simulink model "untitled1"  (R2023a)
settings: Solver=VariableStepAuto  StartTime=0.0  StopTime=30  RelTol=1e-3
settings Model: Creator=Sumeadh  LastModifiedBy=Sumeadh

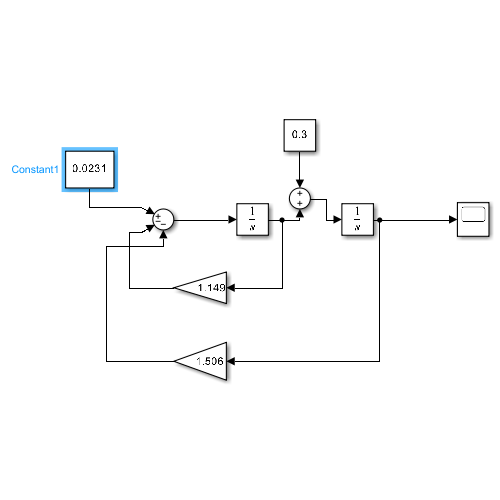
[thumbnail: Simulink's stored preview of the top-level diagram]
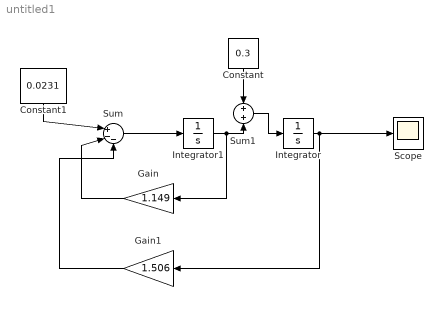
== system untitled1 ==
  Constant : Constant  Value=0.3
  Constant1 : Constant  Value=0.0231
  Gain : Gain  Gain=1.149
  Gain1 : Gain  Gain=1.506
  Integrator : Integrator
  Integrator1 : Integrator
  Scope : Scope
  Sum : Sum  Inputs=|+--
  Sum1 : Sum
  wires:
  Integrator1/1 -> Sum1/2, Gain/1
  Sum/1 -> Integrator1/1
  Integrator/1 -> Gain1/1, Scope/1
  Gain1/1 -> Sum/3
  Gain/1 -> Sum/2
  Constant1/1 -> Sum/1
  Sum1/1 -> Integrator/1
  Constant/1 -> Sum1/1
